simulink model "phm_aug5_powertrain_r2018a"  (R2018a)
settings: Solver=VariableStepAuto  StartTime=0.0  StopTime=750  FixedStep=.01  RelTol=1e-3
InitFcn:
  | addpath fcns;
  | load batteryParams;
  | load motorParams;
  | load ukfBatteryParams;
  | load ukfMotorParams;
undefined symbols (not defined in the file or in its folder): motorParams
libraries: simulink x10
settings Model: Creator=tdarrah  LastModifiedBy=tdarrah
settings SolverCC: ShapePreserveControl=EnableAll  AlgebraicLoopSolver=LineSearch
settings DataIOCC: ReturnWorkspaceOutputs=on
settings SFSimCC: SimUseLocalCustomCode=on
settings RTWCC: RTWUseLocalCustomCode=on

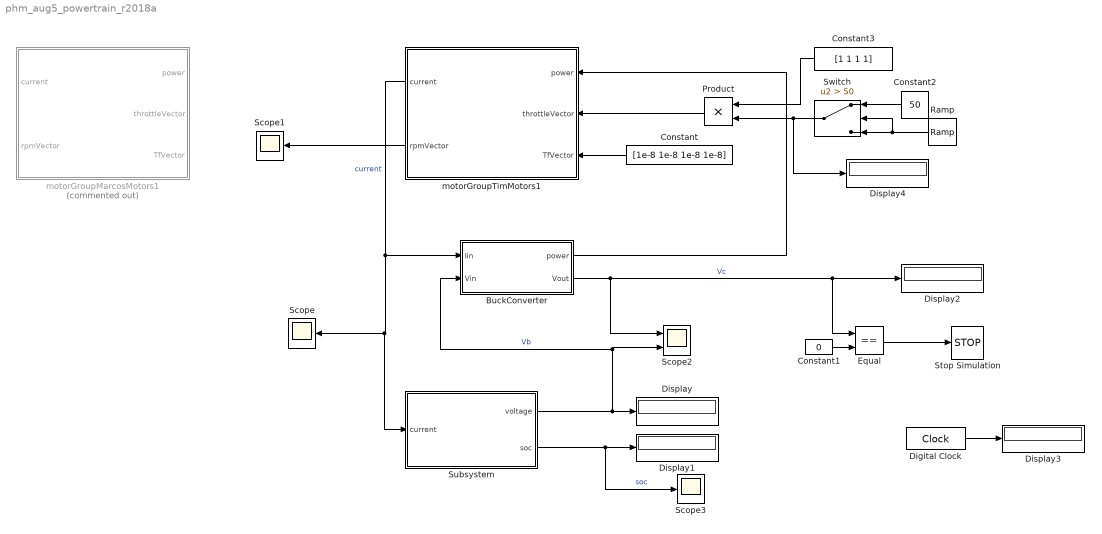
== system phm_aug5_powertrain_r2018a ==
  BuckConverter : Subsystem
  Constant : Constant  Value=[1e-8 1e-8 1e-8 1e-8]
  Constant1 : Constant  Value=0
  Constant2 : Constant  Value=50
  Constant3 : Constant  Value=[1 1 1 1]
  Digital Clock : DigitalClock
      mask Display: disp('Sim Time');
  Display{,1..4} (5 alike) : Display
  Equal : RelationalOperator  Operator===  OutDataTypeStr=boolean  RndMeth=Simplest
  Product : Product
  Ramp : simulink/Sources/Ramp  slope=1  start=0  InitialOutput=0
  Scope : Scope
  Scope1 : Scope
  Scope2 : Scope  NumInputPorts=2
  Scope3 : Scope
  Stop Simulation : Stop
  Subsystem : Subsystem
  Switch : Switch  Criteria=u2 > Threshold  Threshold=50
  motorGroupMarcosMotors1 : Subsystem  Commented=on
  motorGroupTimMotors1 : Subsystem
  wires:
  Subsystem/1(voltage) -> BuckConverter/2(Vin), Scope2/2, Display/1  "Vb"
  Subsystem/2(soc) -> Scope3/1, Display1/1  "soc"
  motorGroupTimMotors1/1(current) -> BuckConverter/1(Iin), Subsystem/1(current), Scope/1  "current"
  BuckConverter/1(power) -> motorGroupTimMotors1/1(power)
  BuckConverter/2(Vout) -> Scope2/1, Equal/1, Display2/1  "Vc"
  Product/1 -> motorGroupTimMotors1/2(throttleVector)
  Constant/1 -> motorGroupTimMotors1/3(TfVector)
  motorGroupTimMotors1/2(rpmVector) -> Scope1/1
  Constant1/1 -> Equal/2
  Equal/1 -> Stop Simulation/1
  Digital Clock/1 -> Display3/1
  Ramp/1 -> Switch/2, Switch/3
  Constant2/1 -> Switch/1
  Constant3/1 -> Product/1
  Switch/1 -> Display4/1, Product/2

== system phm_aug5_powertrain_r2018a/BuckConverter ==
  Iin : Inport
  Vin : Inport  Port=2
  Constant : Constant  Value=0
  Constant2 : Constant  Value=11.4
  If : If  IfExpression=u1 > 10.5
  If Action Subsystem : Subsystem  TreatAsAtomicUnit=on
  If Action Subsystem1 : Subsystem  TreatAsAtomicUnit=on
  Product : Product
  Switch : Switch  Criteria=u2 > Threshold  Threshold=10.5
  power : Outport
  Vout : Outport  Port=2
  wires:
  Product/1 -> power/1
  Iin/1 -> Product/1
  If/1 -> If Action Subsystem/Action
  If/2 -> If Action Subsystem1/Action
  Constant/1 -> If Action Subsystem1/1(In1)
  If Action Subsystem/1(Out1) -> Switch/1
  If Action Subsystem1/1(Out1) -> Switch/3
  Constant2/1 -> If Action Subsystem/1(In1)
  Vin/1 -> Switch/2, If/1
  Switch/1 -> Product/2, Vout/1

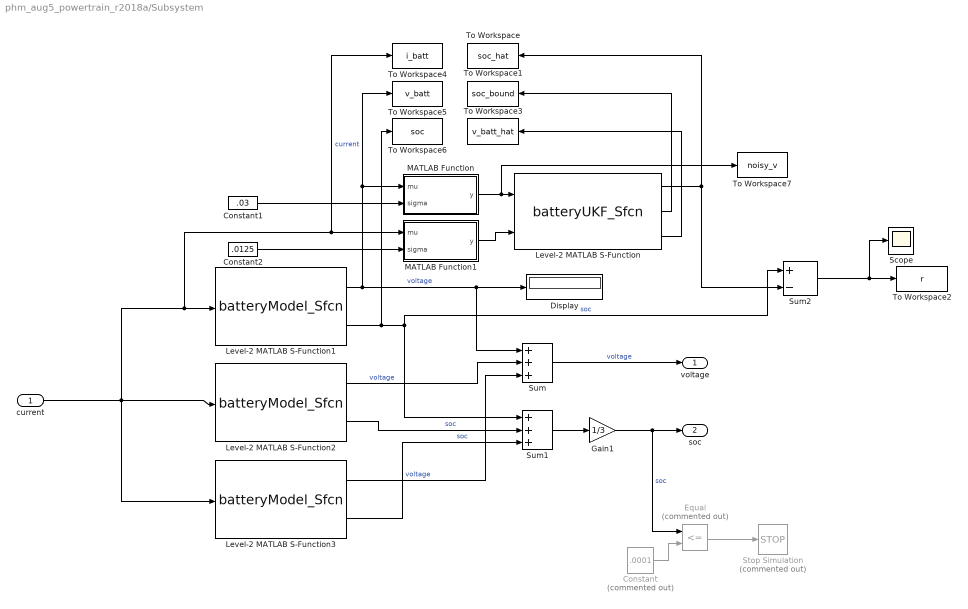
== system phm_aug5_powertrain_r2018a/Subsystem ==
  current : Inport
  Constant : Constant  Commented=on  Value=.0001
  Constant1 : Constant  Value=.03
  Constant2 : Constant  Value=.0125
  Display : Display
  Equal : RelationalOperator  Commented=on  Operator=<=  OutDataTypeStr=boolean  RndMeth=Simplest
  Gain1 : Gain  Gain=1/3
  Level-2 MATLAB S-Function : M-S-Function  FunctionName=batteryUKF_Sfcn  Parameters=batteryParams, batteryParams.dt, ukfBatteryParams
      mask Display:
      | port_label('input', 1, 'voltage');
      | port_label('input', 2, 'current');
      | port_label('output', 1, 'soc_hat');
      | port_label('output', 2, 'soc_bound');
      | port_label('output', 3, 'voltage_hat');
      | 
      | disp("UKF");
  Level-2 MATLAB S-Function1 : M-S-Function  FunctionName=batteryModel_Sfcn  Parameters=batteryParams, batteryParams.dt
      mask Display:
      | port_label('input', 1, 'current');
      | port_label('output', 1, 'voltage');
      | port_label('output', 2, 'soc');
      | 
      | disp("Battery Cell");
  Level-2 MATLAB S-Function2 : M-S-Function  FunctionName=batteryModel_Sfcn  Parameters=batteryParams, batteryParams.dt
      mask Display:
      | port_label('input', 1, 'current');
      | port_label('output', 1, 'voltage');
      | port_label('output', 2, 'soc');
  Level-2 MATLAB S-Function3 : M-S-Function  FunctionName=batteryModel_Sfcn  Parameters=batteryParams, batteryParams.dt
      mask Display:
      | port_label('input', 1, 'current');
      | port_label('output', 1, 'voltage');
      | port_label('output', 2, 'soc');
  MATLAB Function : MATLAB Function  TreatAsAtomicUnit=on
  MATLAB Function1 : MATLAB Function  TreatAsAtomicUnit=on
  Scope : Scope
  Stop Simulation : Stop  Commented=on
  Sum : Sum  Inputs=+++
  Sum1 : Sum  Inputs=+++
  Sum2 : Sum  Inputs=+-
  To Workspace : ToWorkspace  VariableName=soc_hat  SaveFormat=Timeseries  SampleTime=-1
  To Workspace1 : ToWorkspace  VariableName=soc_bound  SaveFormat=Timeseries  SampleTime=-1
  To Workspace2 : ToWorkspace  VariableName=r  SaveFormat=Timeseries  SampleTime=-1
  To Workspace3 : ToWorkspace  VariableName=v_batt_hat  SaveFormat=Timeseries  SampleTime=-1
  To Workspace4 : ToWorkspace  VariableName=i_batt  SaveFormat=Timeseries  SampleTime=-1
  To Workspace5 : ToWorkspace  VariableName=v_batt  SaveFormat=Timeseries  SampleTime=-1
  To Workspace6 : ToWorkspace  VariableName=soc  SaveFormat=Timeseries  SampleTime=-1
  To Workspace7 : ToWorkspace  VariableName=noisy_v  SaveFormat=Timeseries  SampleTime=-1
  voltage : Outport
  soc : Outport  Port=2
  wires:
  Level-2 MATLAB S-Function2/1 -> Sum/2  "voltage"
  Level-2 MATLAB S-Function1/1 -> Display/1, Sum/1, MATLAB Function/1(mu), To Workspace5/1  "voltage"
  Level-2 MATLAB S-Function2/2 -> Sum1/2  "soc"
  Sum1/1 -> Gain1/1
  Gain1/1 -> Equal/1, soc/1  "soc"
  Level-2 MATLAB S-Function1/2 -> To Workspace6/1, Sum2/1, Sum1/1  "soc"
  Level-2 MATLAB S-Function3/2 -> Sum1/3  "soc"
  current/1 -> Level-2 MATLAB S-Function3/1, MATLAB Function1/1(mu), To Workspace4/1, Level-2 MATLAB S-Function1/1, Level-2 MATLAB S-Function2/1  "current"
  Level-2 MATLAB S-Function3/1 -> Sum/3  "voltage"
  Sum/1 -> voltage/1  "voltage"
  Constant/1 -> Equal/2
  Equal/1 -> Stop Simulation/1
  Level-2 MATLAB S-Function/1 -> Sum2/2, To Workspace/1
  Level-2 MATLAB S-Function/2 -> To Workspace1/1
  Sum2/1 -> Scope/1, To Workspace2/1
  Level-2 MATLAB S-Function/3 -> To Workspace3/1
  Constant1/1 -> MATLAB Function/2(sigma)
  MATLAB Function/1(y) -> To Workspace7/1, Level-2 MATLAB S-Function/1
  MATLAB Function1/1(y) -> Level-2 MATLAB S-Function/2
  Constant2/1 -> MATLAB Function1/2(sigma)

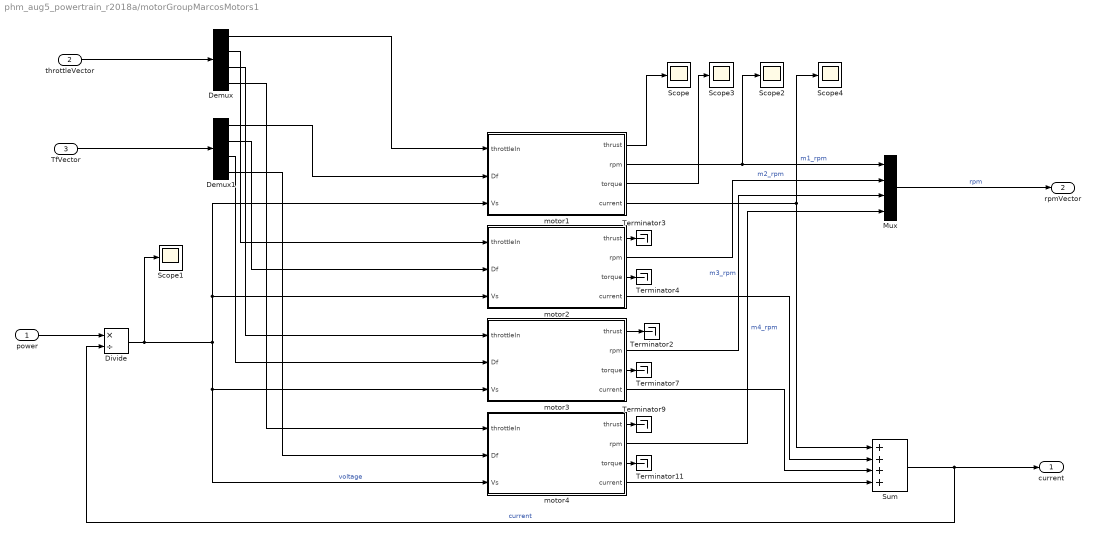
== system phm_aug5_powertrain_r2018a/motorGroupMarcosMotors1 ==
  power : Inport
  throttleVector : Inport  Port=2  PortDimensions=4
  TfVector : Inport  Port=3  PortDimensions=4
  Demux : Demux
  Demux1 : Demux
  Divide : Product  Inputs=*/
  Mux : Mux
  Scope{,1..4} (5 alike) : Scope
  Sum : Sum  Inputs=++++
  Terminator{2..4,7,9,11} (6 alike) : Terminator
  motor1 : Subsystem
  motor2 : Subsystem
  motor3 : Subsystem
  motor4 : Subsystem
  current : Outport
  rpmVector : Outport  Port=2
  wires:
  Demux1/2 -> motor2/2(Df)
  Demux1/4 -> motor4/2(Df)
  Divide/1 -> Scope1/1, motor2/3(Vs), motor1/3(Vs), motor4/3(Vs), motor3/3(Vs)  "voltage"
  Demux1/1 -> motor1/2(Df)
  Sum/1 -> current/1, Divide/2  "current"
  Demux1/3 -> motor3/2(Df)
  motor1/4(current) -> Scope4/1, Sum/1
  power/1 -> Divide/1
  Demux/4 -> motor4/1(throttleIn)
  Demux/3 -> motor3/1(throttleIn)
  Demux/2 -> motor2/1(throttleIn)
  Demux/1 -> motor1/1(throttleIn)
  throttleVector/1 -> Demux/1
  TfVector/1 -> Demux1/1
  motor4/4(current) -> Sum/4
  motor3/4(current) -> Sum/3
  motor2/4(current) -> Sum/2
  motor4/2(rpm) -> Mux/4  "m4_rpm"
  motor3/2(rpm) -> Mux/3  "m3_rpm"
  motor2/2(rpm) -> Mux/2  "m2_rpm"
  motor1/2(rpm) -> Scope2/1, Mux/1  "m1_rpm"
  Mux/1 -> rpmVector/1  "rpm"
  motor1/1(thrust) -> Scope/1
  motor4/3(torque) -> Terminator11/1
  motor1/3(torque) -> Scope3/1
  motor2/3(torque) -> Terminator4/1
  motor3/3(torque) -> Terminator7/1
  motor4/1(thrust) -> Terminator9/1
  motor3/1(thrust) -> Terminator2/1
  motor2/1(thrust) -> Terminator3/1

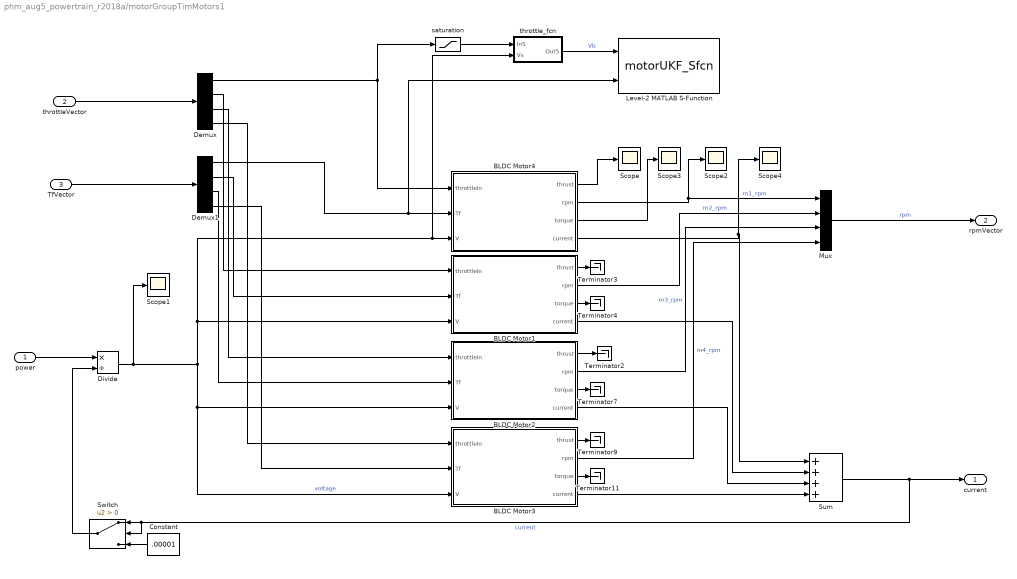
== system phm_aug5_powertrain_r2018a/motorGroupTimMotors1 ==
  power : Inport
  throttleVector : Inport  Port=2  PortDimensions=4
  TfVector : Inport  Port=3  PortDimensions=4
  BLDC Motor1 : Subsystem
  BLDC Motor2 : Subsystem
  BLDC Motor3 : Subsystem
  BLDC Motor4 : Subsystem
  Constant : Constant  Value=.00001
  Demux : Demux
  Demux1 : Demux
  Divide : Product  Inputs=*/
  Level-2 MATLAB S-Function : M-S-Function  FunctionName=motorUKF_Sfcn  Parameters=motorParams, ukfMotorParams
      mask Display:
      | port_label('input', 1, 'voltage');
      | port_label('input', 2, 'friction');
      | port_label('output', 1, 'rpm');
      | port_label('output', 2, 'current');
      | port_label('output', 3, 'torque');
      | port_label('output', 4, 'bounds');
      | disp("Motor UKF");
  Mux : Mux
  Scope{,1..4} (5 alike) : Scope
  Sum : Sum  Inputs=++++
  Switch : Switch  Criteria=u2 > Threshold
  Terminator{2..4,7,9,11} (6 alike) : Terminator
  saturation : Saturate  UpperLimit=100  LowerLimit=0
  throttle_fcn : Subsystem
  current : Outport
  rpmVector : Outport  Port=2
  wires:
  Demux1/2 -> BLDC Motor1/2(Tf)
  Demux1/4 -> BLDC Motor3/2(Tf)
  Divide/1 -> Scope1/1, BLDC Motor1/3(V), throttle_fcn/2(Vs), BLDC Motor4/3(V), BLDC Motor3/3(V), BLDC Motor2/3(V)  "voltage"
  Demux1/1 -> Level-2 MATLAB S-Function/2, BLDC Motor4/2(Tf)
  Sum/1 -> Switch/2, Switch/1, current/1  "current"
  Demux1/3 -> BLDC Motor2/2(Tf)
  BLDC Motor4/4(current) -> Scope4/1, Sum/1
  power/1 -> Divide/1
  Demux/4 -> BLDC Motor3/1(throttleIn)
  Demux/3 -> BLDC Motor2/1(throttleIn)
  Demux/2 -> BLDC Motor1/1(throttleIn)
  Demux/1 -> saturation/1, BLDC Motor4/1(throttleIn)
  throttleVector/1 -> Demux/1
  TfVector/1 -> Demux1/1
  BLDC Motor3/4(current) -> Sum/4
  BLDC Motor2/4(current) -> Sum/3
  BLDC Motor1/4(current) -> Sum/2
  BLDC Motor3/2(rpm) -> Mux/4  "m4_rpm"
  BLDC Motor2/2(rpm) -> Mux/3  "m3_rpm"
  BLDC Motor1/2(rpm) -> Mux/2  "m2_rpm"
  BLDC Motor4/2(rpm) -> Scope2/1, Mux/1  "m1_rpm"
  Mux/1 -> rpmVector/1  "rpm"
  BLDC Motor4/1(thrust) -> Scope/1
  BLDC Motor3/3(torque) -> Terminator11/1
  BLDC Motor4/3(torque) -> Scope3/1
  BLDC Motor1/3(torque) -> Terminator4/1
  BLDC Motor2/3(torque) -> Terminator7/1
  BLDC Motor3/1(thrust) -> Terminator9/1
  BLDC Motor2/1(thrust) -> Terminator2/1
  BLDC Motor1/1(thrust) -> Terminator3/1
  Switch/1 -> Divide/2
  Constant/1 -> Switch/3
  throttle_fcn/1(Out5) -> Level-2 MATLAB S-Function/1  "Vb"
  saturation/1 -> throttle_fcn/1(In5)

== system phm_aug5_powertrain_r2018a/BuckConverter/If Action Subsystem ==
  In1 : Inport
  Action Port : ActionPort
  Out1 : Outport
  wires:
  In1/1 -> Out1/1

== system phm_aug5_powertrain_r2018a/BuckConverter/If Action Subsystem1 ==
  In1 : Inport
  Action Port : ActionPort
  Out1 : Outport
  wires:
  In1/1 -> Out1/1

== system phm_aug5_powertrain_r2018a/motorGroupMarcosMotors1/motor1 ==
  note: Throttle cutoff can simulate the fact that the motor doesn't
      | spin until a minimum throttle point is reached. This introduces
      | a jump discontinuity in low throttle performance.
  note: These saturations model a SIGNAL LIMITATION.
      | Other intentional control saturations might be introduced in the
      | control loop to achieve better stability and consistency.
  throttleIn : Inport
  Df : Inport  Port=2
  Vs : Inport  Port=3
  Scope : Scope
  Signal_Saturation_4 : Saturate  UpperLimit=100  LowerLimit=0
  Throttle To RPM Gain and Cutoff_8 : Subsystem
  motorRotor4 : Subsystem
  thrust : Outport
  rpm : Outport  Port=2
  torque : Outport  Port=3
  current : Outport  Port=4
  wires:
  Throttle To RPM Gain and Cutoff_8/1(Out5) -> motorRotor4/1(V), Scope/1
  motorRotor4/4(current) -> current/1
  motorRotor4/2(rpm) -> rpm/1
  throttleIn/1 -> Signal_Saturation_4/1
  motorRotor4/3(torque) -> torque/1
  motorRotor4/1(thrust) -> thrust/1
  Signal_Saturation_4/1 -> Throttle To RPM Gain and Cutoff_8/1(In5)
  Df/1 -> motorRotor4/2(Df)
  Vs/1 -> Throttle To RPM Gain and Cutoff_8/2(Vs)

== system phm_aug5_powertrain_r2018a/motorGroupMarcosMotors1/motor2 ==
  note: Throttle cutoff can simulate the fact that the motor doesn't
      | spin until a minimum throttle point is reached. This introduces
      | a jump discontinuity in low throttle performance.
  note: These saturations model a SIGNAL LIMITATION.
      | Other intentional control saturations might be introduced in the
      | control loop to achieve better stability and consistency.
  throttleIn : Inport
  Df : Inport  Port=2
  Vs : Inport  Port=3
  Scope : Scope
  Signal_Saturation_4 : Saturate  UpperLimit=100  LowerLimit=0
  Throttle To RPM Gain and Cutoff_8 : Subsystem
  motorRotor4 : Subsystem
  thrust : Outport
  rpm : Outport  Port=2
  torque : Outport  Port=3
  current : Outport  Port=4
  wires:
  Throttle To RPM Gain and Cutoff_8/1(Out5) -> motorRotor4/1(V), Scope/1
  motorRotor4/4(current) -> current/1
  motorRotor4/2(rpm) -> rpm/1
  throttleIn/1 -> Signal_Saturation_4/1
  motorRotor4/3(torque) -> torque/1
  motorRotor4/1(thrust) -> thrust/1
  Signal_Saturation_4/1 -> Throttle To RPM Gain and Cutoff_8/1(In5)
  Df/1 -> motorRotor4/2(Df)
  Vs/1 -> Throttle To RPM Gain and Cutoff_8/2(Vs)

== system phm_aug5_powertrain_r2018a/motorGroupMarcosMotors1/motor3 ==
  note: Throttle cutoff can simulate the fact that the motor doesn't
      | spin until a minimum throttle point is reached. This introduces
      | a jump discontinuity in low throttle performance.
  note: These saturations model a SIGNAL LIMITATION.
      | Other intentional control saturations might be introduced in the
      | control loop to achieve better stability and consistency.
  throttleIn : Inport
  Df : Inport  Port=2
  Vs : Inport  Port=3
  Scope : Scope
  Signal_Saturation_4 : Saturate  UpperLimit=100  LowerLimit=0
  Throttle To RPM Gain and Cutoff_8 : Subsystem
  motorRotor4 : Subsystem
  thrust : Outport
  rpm : Outport  Port=2
  torque : Outport  Port=3
  current : Outport  Port=4
  wires:
  Throttle To RPM Gain and Cutoff_8/1(Out5) -> motorRotor4/1(V), Scope/1
  motorRotor4/4(current) -> current/1
  motorRotor4/2(rpm) -> rpm/1
  throttleIn/1 -> Signal_Saturation_4/1
  motorRotor4/3(torque) -> torque/1
  motorRotor4/1(thrust) -> thrust/1
  Signal_Saturation_4/1 -> Throttle To RPM Gain and Cutoff_8/1(In5)
  Df/1 -> motorRotor4/2(Df)
  Vs/1 -> Throttle To RPM Gain and Cutoff_8/2(Vs)

== system phm_aug5_powertrain_r2018a/motorGroupMarcosMotors1/motor4 ==
  note: Throttle cutoff can simulate the fact that the motor doesn't
      | spin until a minimum throttle point is reached. This introduces
      | a jump discontinuity in low throttle performance.
  note: These saturations model a SIGNAL LIMITATION.
      | Other intentional control saturations might be introduced in the
      | control loop to achieve better stability and consistency.
  throttleIn : Inport
  Df : Inport  Port=2
  Vs : Inport  Port=3
  Scope : Scope
  Signal_Saturation_4 : Saturate  UpperLimit=100  LowerLimit=0
  Throttle To RPM Gain and Cutoff_8 : Subsystem
  motorRotor4 : Subsystem
  thrust : Outport
  rpm : Outport  Port=2
  torque : Outport  Port=3
  current : Outport  Port=4
  wires:
  Throttle To RPM Gain and Cutoff_8/1(Out5) -> motorRotor4/1(V), Scope/1
  motorRotor4/4(current) -> current/1
  motorRotor4/2(rpm) -> rpm/1
  throttleIn/1 -> Signal_Saturation_4/1
  motorRotor4/3(torque) -> torque/1
  motorRotor4/1(thrust) -> thrust/1
  Signal_Saturation_4/1 -> Throttle To RPM Gain and Cutoff_8/1(In5)
  Df/1 -> motorRotor4/2(Df)
  Vs/1 -> Throttle To RPM Gain and Cutoff_8/2(Vs)

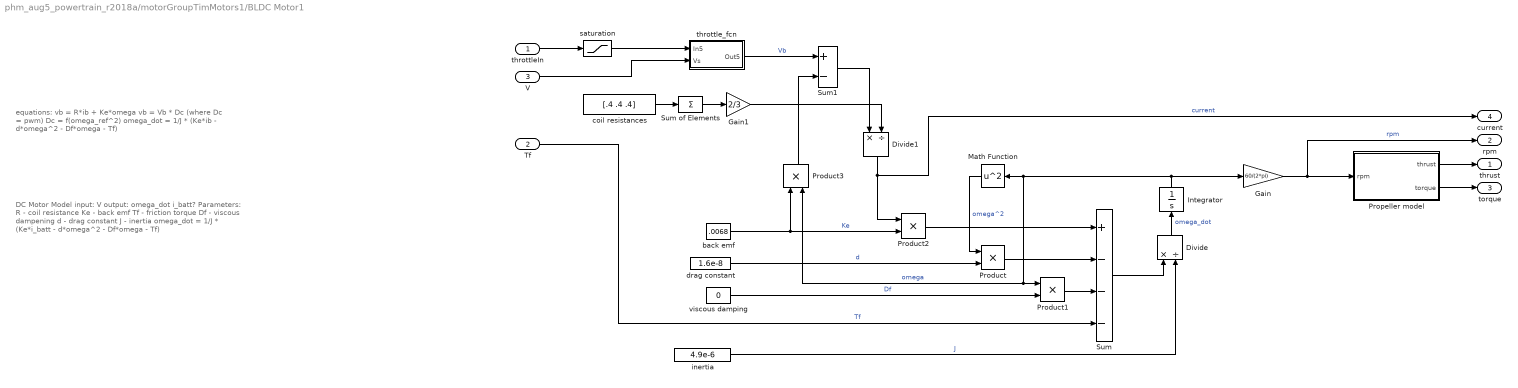
== system phm_aug5_powertrain_r2018a/motorGroupTimMotors1/BLDC Motor1 ==
  note: DC Motor Model
      |
      | input:
      | V
      |
      | output:
      | omega_dot
      | i_batt?
      |
      |
      | Parameters:
      | R   - coil resistance
      | Ke - back emf
      | Tf  - friction torque
      | Df  - viscous dampening
      | d   - drag constant
      | J   - inertia
      |
      | omega_dot = 1/J * (Ke*i_batt - d*omega^2 - Df*omega - Tf)
  note: equations:
      |
      | vb = R*ib + Ke*omega
      | vb = Vb * Dc  (where Dc = pwm)
      | Dc = f(omega_ref^2)
      |
      | omega_dot = 1/J * (Ke*ib - d*omega^2 - Df*omega - Tf)
  throttleIn : Inport
  Tf : Inport  Port=2
  V : Inport  Port=3
  Divide : Product  Inputs=*/
  Divide1 : Product  Inputs=*/
  Gain : Gain  Gain=60/(2*pi)
  Gain1 : Gain  Gain=2/3
  Integrator : Integrator
  Math Function : Math  Operator=square  SaturateOnIntegerOverflow=on
  Product{,1..3} (4 alike) : Product
  "Propeller model " : MATLAB Function  TreatAsAtomicUnit=on
  Sum : Sum  Inputs=+---
  Sum of Elements : Sum  Inputs=+
  Sum1 : Sum  Inputs=+-
  back emf : Constant  Value=.0068
  coil resistances : Constant  Value=[.4 .4 .4]
  drag constant : Constant  Value=1.6e-8
  inertia : Constant  Value=4.9e-6
  saturation : Saturate  UpperLimit=100  LowerLimit=0
  throttle_fcn : Subsystem
  viscous damping : Constant  Value=0
  thrust : Outport
  rpm : Outport  Port=2
  torque : Outport  Port=3
  current : Outport  Port=4
  wires:
  Divide/1 -> Integrator/1  "omega_dot"
  Integrator/1 -> Gain/1, Math Function/1, Product1/1, Product3/2  "omega"
  Gain/1 -> "Propeller model "/1(rpm), rpm/1  "rpm"
  inertia/1 -> Divide/2  "J"
  drag constant/1 -> Product/2  "d"
  Math Function/1 -> Product/1  "omega^2"
  viscous damping/1 -> Product1/2  "Df"
  Tf/1 -> Sum/4  "Tf"
  back emf/1 -> Product3/1, Product2/2  "Ke"
  Product2/1 -> Sum/1
  Divide1/1 -> current/1, Product2/1  "current"
  V/1 -> throttle_fcn/2(Vs)
  Product3/1 -> Sum1/2
  Sum1/1 -> Divide1/1
  Gain1/1 -> Divide1/2
  "Propeller model "/1(thrust) -> thrust/1
  "Propeller model "/2(torque) -> torque/1
  Product1/1 -> Sum/3
  Product/1 -> Sum/2
  Sum/1 -> Divide/1
  coil resistances/1 -> Sum of Elements/1
  Sum of Elements/1 -> Gain1/1
  throttleIn/1 -> saturation/1
  throttle_fcn/1(Out5) -> Sum1/1  "Vb"
  saturation/1 -> throttle_fcn/1(In5)

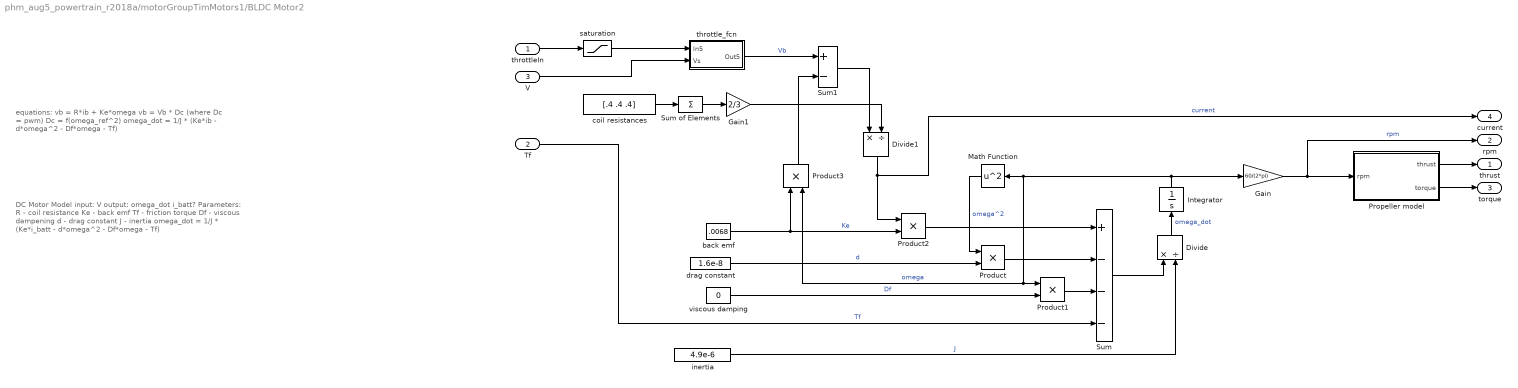
== system phm_aug5_powertrain_r2018a/motorGroupTimMotors1/BLDC Motor2 ==
  note: DC Motor Model
      |
      | input:
      | V
      |
      | output:
      | omega_dot
      | i_batt?
      |
      |
      | Parameters:
      | R   - coil resistance
      | Ke - back emf
      | Tf  - friction torque
      | Df  - viscous dampening
      | d   - drag constant
      | J   - inertia
      |
      | omega_dot = 1/J * (Ke*i_batt - d*omega^2 - Df*omega - Tf)
  note: equations:
      |
      | vb = R*ib + Ke*omega
      | vb = Vb * Dc  (where Dc = pwm)
      | Dc = f(omega_ref^2)
      |
      | omega_dot = 1/J * (Ke*ib - d*omega^2 - Df*omega - Tf)
  throttleIn : Inport
  Tf : Inport  Port=2
  V : Inport  Port=3
  Divide : Product  Inputs=*/
  Divide1 : Product  Inputs=*/
  Gain : Gain  Gain=60/(2*pi)
  Gain1 : Gain  Gain=2/3
  Integrator : Integrator
  Math Function : Math  Operator=square  SaturateOnIntegerOverflow=on
  Product{,1..3} (4 alike) : Product
  "Propeller model " : MATLAB Function  TreatAsAtomicUnit=on
  Sum : Sum  Inputs=+---
  Sum of Elements : Sum  Inputs=+
  Sum1 : Sum  Inputs=+-
  back emf : Constant  Value=.0068
  coil resistances : Constant  Value=[.4 .4 .4]
  drag constant : Constant  Value=1.6e-8
  inertia : Constant  Value=4.9e-6
  saturation : Saturate  UpperLimit=100  LowerLimit=0
  throttle_fcn : Subsystem
  viscous damping : Constant  Value=0
  thrust : Outport
  rpm : Outport  Port=2
  torque : Outport  Port=3
  current : Outport  Port=4
  wires:
  Divide/1 -> Integrator/1  "omega_dot"
  Integrator/1 -> Gain/1, Math Function/1, Product1/1, Product3/2  "omega"
  Gain/1 -> "Propeller model "/1(rpm), rpm/1  "rpm"
  inertia/1 -> Divide/2  "J"
  drag constant/1 -> Product/2  "d"
  Math Function/1 -> Product/1  "omega^2"
  viscous damping/1 -> Product1/2  "Df"
  Tf/1 -> Sum/4  "Tf"
  back emf/1 -> Product3/1, Product2/2  "Ke"
  Product2/1 -> Sum/1
  Divide1/1 -> current/1, Product2/1  "current"
  V/1 -> throttle_fcn/2(Vs)
  Product3/1 -> Sum1/2
  Sum1/1 -> Divide1/1
  Gain1/1 -> Divide1/2
  "Propeller model "/1(thrust) -> thrust/1
  "Propeller model "/2(torque) -> torque/1
  Product1/1 -> Sum/3
  Product/1 -> Sum/2
  Sum/1 -> Divide/1
  coil resistances/1 -> Sum of Elements/1
  Sum of Elements/1 -> Gain1/1
  throttleIn/1 -> saturation/1
  throttle_fcn/1(Out5) -> Sum1/1  "Vb"
  saturation/1 -> throttle_fcn/1(In5)

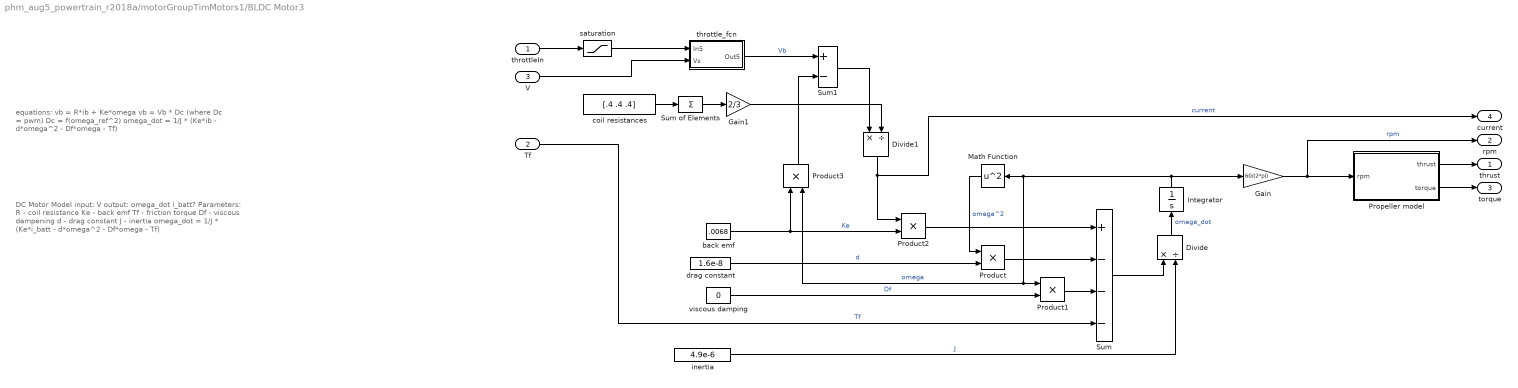
== system phm_aug5_powertrain_r2018a/motorGroupTimMotors1/BLDC Motor3 ==
  note: DC Motor Model
      |
      | input:
      | V
      |
      | output:
      | omega_dot
      | i_batt?
      |
      |
      | Parameters:
      | R   - coil resistance
      | Ke - back emf
      | Tf  - friction torque
      | Df  - viscous dampening
      | d   - drag constant
      | J   - inertia
      |
      | omega_dot = 1/J * (Ke*i_batt - d*omega^2 - Df*omega - Tf)
  note: equations:
      |
      | vb = R*ib + Ke*omega
      | vb = Vb * Dc  (where Dc = pwm)
      | Dc = f(omega_ref^2)
      |
      | omega_dot = 1/J * (Ke*ib - d*omega^2 - Df*omega - Tf)
  throttleIn : Inport
  Tf : Inport  Port=2
  V : Inport  Port=3
  Divide : Product  Inputs=*/
  Divide1 : Product  Inputs=*/
  Gain : Gain  Gain=60/(2*pi)
  Gain1 : Gain  Gain=2/3
  Integrator : Integrator
  Math Function : Math  Operator=square  SaturateOnIntegerOverflow=on
  Product{,1..3} (4 alike) : Product
  "Propeller model " : MATLAB Function  TreatAsAtomicUnit=on
  Sum : Sum  Inputs=+---
  Sum of Elements : Sum  Inputs=+
  Sum1 : Sum  Inputs=+-
  back emf : Constant  Value=.0068
  coil resistances : Constant  Value=[.4 .4 .4]
  drag constant : Constant  Value=1.6e-8
  inertia : Constant  Value=4.9e-6
  saturation : Saturate  UpperLimit=100  LowerLimit=0
  throttle_fcn : Subsystem
  viscous damping : Constant  Value=0
  thrust : Outport
  rpm : Outport  Port=2
  torque : Outport  Port=3
  current : Outport  Port=4
  wires:
  Divide/1 -> Integrator/1  "omega_dot"
  Integrator/1 -> Gain/1, Math Function/1, Product1/1, Product3/2  "omega"
  Gain/1 -> "Propeller model "/1(rpm), rpm/1  "rpm"
  inertia/1 -> Divide/2  "J"
  drag constant/1 -> Product/2  "d"
  Math Function/1 -> Product/1  "omega^2"
  viscous damping/1 -> Product1/2  "Df"
  Tf/1 -> Sum/4  "Tf"
  back emf/1 -> Product3/1, Product2/2  "Ke"
  Product2/1 -> Sum/1
  Divide1/1 -> current/1, Product2/1  "current"
  V/1 -> throttle_fcn/2(Vs)
  Product3/1 -> Sum1/2
  Sum1/1 -> Divide1/1
  Gain1/1 -> Divide1/2
  "Propeller model "/1(thrust) -> thrust/1
  "Propeller model "/2(torque) -> torque/1
  Product1/1 -> Sum/3
  Product/1 -> Sum/2
  Sum/1 -> Divide/1
  coil resistances/1 -> Sum of Elements/1
  Sum of Elements/1 -> Gain1/1
  throttleIn/1 -> saturation/1
  throttle_fcn/1(Out5) -> Sum1/1  "Vb"
  saturation/1 -> throttle_fcn/1(In5)

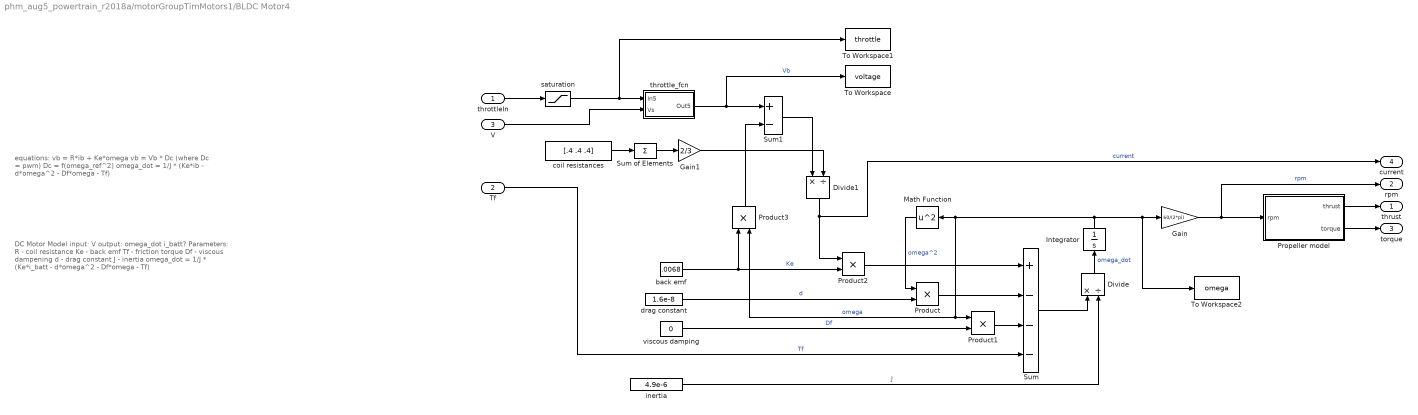
== system phm_aug5_powertrain_r2018a/motorGroupTimMotors1/BLDC Motor4 ==
  note: DC Motor Model
      |
      | input:
      | V
      |
      | output:
      | omega_dot
      | i_batt?
      |
      |
      | Parameters:
      | R   - coil resistance
      | Ke - back emf
      | Tf  - friction torque
      | Df  - viscous dampening
      | d   - drag constant
      | J   - inertia
      |
      | omega_dot = 1/J * (Ke*i_batt - d*omega^2 - Df*omega - Tf)
  note: equations:
      |
      | vb = R*ib + Ke*omega
      | vb = Vb * Dc  (where Dc = pwm)
      | Dc = f(omega_ref^2)
      |
      | omega_dot = 1/J * (Ke*ib - d*omega^2 - Df*omega - Tf)
  throttleIn : Inport
  Tf : Inport  Port=2
  V : Inport  Port=3
  Divide : Product  Inputs=*/
  Divide1 : Product  Inputs=*/
  Gain : Gain  Gain=60/(2*pi)
  Gain1 : Gain  Gain=2/3
  Integrator : Integrator
  Math Function : Math  Operator=square  SaturateOnIntegerOverflow=on
  Product{,1..3} (4 alike) : Product
  "Propeller model " : MATLAB Function  TreatAsAtomicUnit=on
  Sum : Sum  Inputs=+---
  Sum of Elements : Sum  Inputs=+
  Sum1 : Sum  Inputs=+-
  To Workspace : ToWorkspace  VariableName=voltage  SaveFormat=Timeseries  SampleTime=-1
  To Workspace1 : ToWorkspace  VariableName=throttle  SaveFormat=Timeseries  SampleTime=-1
  To Workspace2 : ToWorkspace  VariableName=omega  SaveFormat=Timeseries  SampleTime=-1
  back emf : Constant  Value=.0068
  coil resistances : Constant  Value=[.4 .4 .4]
  drag constant : Constant  Value=1.6e-8
  inertia : Constant  Value=4.9e-6
  saturation : Saturate  UpperLimit=100  LowerLimit=0
  throttle_fcn : Subsystem
  viscous damping : Constant  Value=0
  thrust : Outport
  rpm : Outport  Port=2
  torque : Outport  Port=3
  current : Outport  Port=4
  wires:
  Divide/1 -> Integrator/1  "omega_dot"
  Integrator/1 -> To Workspace2/1, Gain/1, Math Function/1, Product1/1, Product3/2  "omega"
  Gain/1 -> "Propeller model "/1(rpm), rpm/1  "rpm"
  inertia/1 -> Divide/2  "J"
  drag constant/1 -> Product/2  "d"
  Math Function/1 -> Product/1  "omega^2"
  viscous damping/1 -> Product1/2  "Df"
  Tf/1 -> Sum/4  "Tf"
  back emf/1 -> Product3/1, Product2/2  "Ke"
  Product2/1 -> Sum/1
  Divide1/1 -> current/1, Product2/1  "current"
  V/1 -> throttle_fcn/2(Vs)
  Product3/1 -> Sum1/2
  Sum1/1 -> Divide1/1
  Gain1/1 -> Divide1/2
  "Propeller model "/1(thrust) -> thrust/1
  "Propeller model "/2(torque) -> torque/1
  Product1/1 -> Sum/3
  Product/1 -> Sum/2
  Sum/1 -> Divide/1
  coil resistances/1 -> Sum of Elements/1
  Sum of Elements/1 -> Gain1/1
  throttleIn/1 -> saturation/1
  throttle_fcn/1(Out5) -> To Workspace/1, Sum1/1  "Vb"
  saturation/1 -> To Workspace1/1, throttle_fcn/1(In5)

== system phm_aug5_powertrain_r2018a/motorGroupTimMotors1/throttle_fcn ==
  note: Output equals linearly scaled RPM
      | for given throttle input if throttle input >=Throttle Cuttoff (minThr)
      | else output is zero.
  In5 : Inport
  Vs : Inport  Port=2
  Gain : Gain  Gain=.01
  Minimum Throttle Cutoff : simulink/Logic and Bit Operations/Compare To Constant  relop=>=  const=5  OutDataTypeStr=uint8
  Product : Product
  Product2 : Product
  Out5 : Outport
  wires:
  Minimum Throttle Cutoff/1 -> Product/2
  Product/1 -> Out5/1
  In5/1 -> Gain/1, Minimum Throttle Cutoff/1
  Gain/1 -> Product2/2
  Product2/1 -> Product/1
  Vs/1 -> Product2/1

== system phm_aug5_powertrain_r2018a/motorGroupMarcosMotors1/motor1/Throttle To RPM Gain and Cutoff_8 ==
  note: Output equals linearly scaled RPM
      | for given throttle input if throttle input >=Throttle Cuttoff (minThr)
      | else output is zero.
  In5 : Inport
  Vs : Inport  Port=2
  Gain : Gain  Gain=.01
  Minimum Throttle Cutoff : simulink/Logic and Bit Operations/Compare To Constant  relop=>=  const=5  OutDataTypeStr=uint8
  Product : Product
  Product2 : Product
  Out5 : Outport
  wires:
  Minimum Throttle Cutoff/1 -> Product/2
  Product/1 -> Out5/1
  In5/1 -> Gain/1, Minimum Throttle Cutoff/1
  Gain/1 -> Product2/2
  Product2/1 -> Product/1
  Vs/1 -> Product2/1

== system phm_aug5_powertrain_r2018a/motorGroupMarcosMotors1/motor1/motorRotor4 ==
  V : Inport
  Df : Inport  Port=2
  Electrical part : Subsystem
  Mechanical part : Subsystem
  thrust : Outport
  rpm : Outport  Port=2
  torque : Outport  Port=3
  current : Outport  Port=4
  wires:
  V/1 -> Electrical part/1(Vin)
  Mechanical part/2(Thrust) -> thrust/1
  Electrical part/1(Electrical Torque) -> Mechanical part/2(Electrical Torque)
  Mechanical part/4(Torque) -> torque/1
  Mechanical part/1(w angular speed) -> Electrical part/2(w angular speed)
  Df/1 -> Mechanical part/1(dynamicFriction)
  Electrical part/2(current) -> current/1
  Mechanical part/3(rpm) -> rpm/1

== system phm_aug5_powertrain_r2018a/motorGroupMarcosMotors1/motor2/Throttle To RPM Gain and Cutoff_8 ==
  note: Output equals linearly scaled RPM
      | for given throttle input if throttle input >=Throttle Cuttoff (minThr)
      | else output is zero.
  In5 : Inport
  Vs : Inport  Port=2
  Gain : Gain  Gain=.01
  Minimum Throttle Cutoff : simulink/Logic and Bit Operations/Compare To Constant  relop=>=  const=5  OutDataTypeStr=uint8
  Product : Product
  Product2 : Product
  Out5 : Outport
  wires:
  Minimum Throttle Cutoff/1 -> Product/2
  Product/1 -> Out5/1
  In5/1 -> Gain/1, Minimum Throttle Cutoff/1
  Gain/1 -> Product2/2
  Product2/1 -> Product/1
  Vs/1 -> Product2/1

== system phm_aug5_powertrain_r2018a/motorGroupMarcosMotors1/motor2/motorRotor4 ==
  V : Inport
  Df : Inport  Port=2
  Electrical part : Subsystem
  Mechanical part : Subsystem
  thrust : Outport
  rpm : Outport  Port=2
  torque : Outport  Port=3
  current : Outport  Port=4
  wires:
  V/1 -> Electrical part/1(Vin)
  Mechanical part/2(Thrust) -> thrust/1
  Electrical part/1(Electrical Torque) -> Mechanical part/2(Electrical Torque)
  Mechanical part/4(Torque) -> torque/1
  Mechanical part/1(w angular speed) -> Electrical part/2(w angular speed)
  Df/1 -> Mechanical part/1(dynamicFriction)
  Electrical part/2(current) -> current/1
  Mechanical part/3(rpm) -> rpm/1

== system phm_aug5_powertrain_r2018a/motorGroupMarcosMotors1/motor3/Throttle To RPM Gain and Cutoff_8 ==
  note: Output equals linearly scaled RPM
      | for given throttle input if throttle input >=Throttle Cuttoff (minThr)
      | else output is zero.
  In5 : Inport
  Vs : Inport  Port=2
  Gain : Gain  Gain=.01
  Minimum Throttle Cutoff : simulink/Logic and Bit Operations/Compare To Constant  relop=>=  const=5  OutDataTypeStr=uint8
  Product : Product
  Product2 : Product
  Out5 : Outport
  wires:
  Minimum Throttle Cutoff/1 -> Product/2
  Product/1 -> Out5/1
  In5/1 -> Gain/1, Minimum Throttle Cutoff/1
  Gain/1 -> Product2/2
  Product2/1 -> Product/1
  Vs/1 -> Product2/1

== system phm_aug5_powertrain_r2018a/motorGroupMarcosMotors1/motor3/motorRotor4 ==
  V : Inport
  Df : Inport  Port=2
  Electrical part : Subsystem
  Mechanical part : Subsystem
  thrust : Outport
  rpm : Outport  Port=2
  torque : Outport  Port=3
  current : Outport  Port=4
  wires:
  V/1 -> Electrical part/1(Vin)
  Mechanical part/2(Thrust) -> thrust/1
  Electrical part/1(Electrical Torque) -> Mechanical part/2(Electrical Torque)
  Mechanical part/4(Torque) -> torque/1
  Mechanical part/1(w angular speed) -> Electrical part/2(w angular speed)
  Df/1 -> Mechanical part/1(dynamicFriction)
  Electrical part/2(current) -> current/1
  Mechanical part/3(rpm) -> rpm/1

== system phm_aug5_powertrain_r2018a/motorGroupMarcosMotors1/motor4/Throttle To RPM Gain and Cutoff_8 ==
  note: Output equals linearly scaled RPM
      | for given throttle input if throttle input >=Throttle Cuttoff (minThr)
      | else output is zero.
  In5 : Inport
  Vs : Inport  Port=2
  Gain : Gain  Gain=.01
  Minimum Throttle Cutoff : simulink/Logic and Bit Operations/Compare To Constant  relop=>=  const=5  OutDataTypeStr=uint8
  Product : Product
  Product2 : Product
  Out5 : Outport
  wires:
  Minimum Throttle Cutoff/1 -> Product/2
  Product/1 -> Out5/1
  In5/1 -> Gain/1, Minimum Throttle Cutoff/1
  Gain/1 -> Product2/2
  Product2/1 -> Product/1
  Vs/1 -> Product2/1

== system phm_aug5_powertrain_r2018a/motorGroupMarcosMotors1/motor4/motorRotor4 ==
  V : Inport
  Df : Inport  Port=2
  Electrical part : Subsystem
  Mechanical part : Subsystem
  thrust : Outport
  rpm : Outport  Port=2
  torque : Outport  Port=3
  current : Outport  Port=4
  wires:
  V/1 -> Electrical part/1(Vin)
  Mechanical part/2(Thrust) -> thrust/1
  Electrical part/1(Electrical Torque) -> Mechanical part/2(Electrical Torque)
  Mechanical part/4(Torque) -> torque/1
  Mechanical part/1(w angular speed) -> Electrical part/2(w angular speed)
  Df/1 -> Mechanical part/1(dynamicFriction)
  Electrical part/2(current) -> current/1
  Mechanical part/3(rpm) -> rpm/1

== system phm_aug5_powertrain_r2018a/motorGroupTimMotors1/BLDC Motor1/throttle_fcn ==
  note: Output equals linearly scaled RPM
      | for given throttle input if throttle input >=Throttle Cuttoff (minThr)
      | else output is zero.
  In5 : Inport
  Vs : Inport  Port=2
  Gain : Gain  Gain=.01
  Minimum Throttle Cutoff : simulink/Logic and Bit Operations/Compare To Constant  relop=>=  const=5  OutDataTypeStr=uint8
  Product : Product
  Product2 : Product  OutDataTypeStr=double
  Out5 : Outport
  wires:
  Minimum Throttle Cutoff/1 -> Product/2
  Product/1 -> Out5/1
  In5/1 -> Gain/1, Minimum Throttle Cutoff/1
  Gain/1 -> Product2/2
  Product2/1 -> Product/1
  Vs/1 -> Product2/1

== system phm_aug5_powertrain_r2018a/motorGroupTimMotors1/BLDC Motor2/throttle_fcn ==
  note: Output equals linearly scaled RPM
      | for given throttle input if throttle input >=Throttle Cuttoff (minThr)
      | else output is zero.
  In5 : Inport
  Vs : Inport  Port=2
  Gain : Gain  Gain=.01
  Minimum Throttle Cutoff : simulink/Logic and Bit Operations/Compare To Constant  relop=>=  const=5  OutDataTypeStr=uint8
  Product : Product
  Product2 : Product  OutDataTypeStr=double
  Out5 : Outport
  wires:
  Minimum Throttle Cutoff/1 -> Product/2
  Product/1 -> Out5/1
  In5/1 -> Gain/1, Minimum Throttle Cutoff/1
  Gain/1 -> Product2/2
  Product2/1 -> Product/1
  Vs/1 -> Product2/1

== system phm_aug5_powertrain_r2018a/motorGroupTimMotors1/BLDC Motor3/throttle_fcn ==
  note: Output equals linearly scaled RPM
      | for given throttle input if throttle input >=Throttle Cuttoff (minThr)
      | else output is zero.
  In5 : Inport
  Vs : Inport  Port=2
  Gain : Gain  Gain=.01
  Minimum Throttle Cutoff : simulink/Logic and Bit Operations/Compare To Constant  relop=>=  const=5  OutDataTypeStr=uint8
  Product : Product
  Product2 : Product  OutDataTypeStr=double
  Out5 : Outport
  wires:
  Minimum Throttle Cutoff/1 -> Product/2
  Product/1 -> Out5/1
  In5/1 -> Gain/1, Minimum Throttle Cutoff/1
  Gain/1 -> Product2/2
  Product2/1 -> Product/1
  Vs/1 -> Product2/1

== system phm_aug5_powertrain_r2018a/motorGroupTimMotors1/BLDC Motor4/throttle_fcn ==
  note: Output equals linearly scaled RPM
      | for given throttle input if throttle input >=Throttle Cuttoff (minThr)
      | else output is zero.
  In5 : Inport
  Vs : Inport  Port=2
  Gain : Gain  Gain=.01
  Minimum Throttle Cutoff : simulink/Logic and Bit Operations/Compare To Constant  relop=>=  const=5  OutDataTypeStr=uint8
  Product : Product
  Product2 : Product  OutDataTypeStr=double
  Out5 : Outport
  wires:
  Minimum Throttle Cutoff/1 -> Product/2
  Product/1 -> Out5/1
  In5/1 -> Gain/1, Minimum Throttle Cutoff/1
  Gain/1 -> Product2/2
  Product2/1 -> Product/1
  Vs/1 -> Product2/1

== system phm_aug5_powertrain_r2018a/motorGroupMarcosMotors1/motor1/motorRotor4/Electrical part ==
  Vin : Inport
  w angular speed : Inport  Port=2
  1/R : Gain  Gain=1/motorParams.Req
  Ke (Torque constant)1 : Gain  Gain=motorParams.Ke_eq
  Kt (Torque constant) Kt=Ke for an ideal square wave motor : Gain  Gain=motorParams.Ke_eq
  Sum : Sum  Inputs=|+-
  Electrical Torque : Outport
  current : Outport  Port=2
  wires:
  1/R/1 -> current/1, Kt (Torque constant) Kt=Ke for an ideal square wave motor/1  "current i"
  Sum/1 -> 1/R/1
  Kt (Torque constant) Kt=Ke for an ideal square wave motor/1 -> Electrical Torque/1
  Ke (Torque constant)1/1 -> Sum/2
  Vin/1 -> Sum/1
  w angular speed/1 -> Ke (Torque constant)1/1

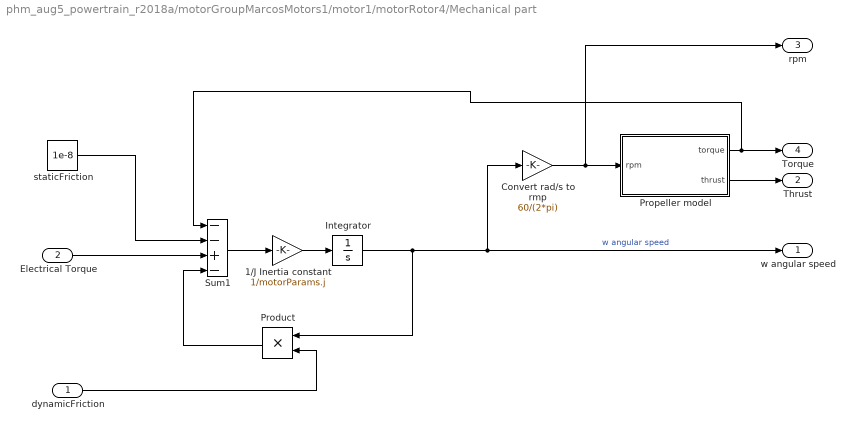
== system phm_aug5_powertrain_r2018a/motorGroupMarcosMotors1/motor1/motorRotor4/Mechanical part ==
  dynamicFriction : Inport
  Electrical Torque : Inport  Port=2
  1/J Inertia constant : Gain  Gain=1/motorParams.j
  Convert rad/s to rmp : Gain  Gain=60/(2*pi)
  Integrator : Integrator  InitialCondition=419
  Product : Product
  "Propeller model " : MATLAB Function  TreatAsAtomicUnit=on
  Sum1 : Sum  Inputs=--+-
  staticFriction : Constant  Value=1e-8
  w angular speed : Outport
  Thrust : Outport  Port=2
  rpm : Outport  Port=3
  Torque : Outport  Port=4
  wires:
  "Propeller model "/1(torque) -> Sum1/1, Torque/1
  1/J Inertia constant/1 -> Integrator/1
  dynamicFriction/1 -> Product/2
  Product/1 -> Sum1/4
  Integrator/1 -> Product/1, w angular speed/1, Convert rad/s to rmp/1  "w angular speed"
  Sum1/1 -> 1/J Inertia constant/1
  Electrical Torque/1 -> Sum1/3
  Convert rad/s to rmp/1 -> rpm/1, "Propeller model "/1(rpm)
  "Propeller model "/2(thrust) -> Thrust/1
  staticFriction/1 -> Sum1/2

== system phm_aug5_powertrain_r2018a/motorGroupMarcosMotors1/motor2/motorRotor4/Electrical part ==
  Vin : Inport
  w angular speed : Inport  Port=2
  1/R : Gain  Gain=1/motorParams.Req
  Ke (Torque constant)1 : Gain  Gain=motorParams.Ke_eq
  Kt (Torque constant) Kt=Ke for an ideal square wave motor : Gain  Gain=motorParams.Ke_eq
  Sum : Sum  Inputs=|+-
  Electrical Torque : Outport
  current : Outport  Port=2
  wires:
  1/R/1 -> current/1, Kt (Torque constant) Kt=Ke for an ideal square wave motor/1  "current i"
  Sum/1 -> 1/R/1
  Kt (Torque constant) Kt=Ke for an ideal square wave motor/1 -> Electrical Torque/1
  Ke (Torque constant)1/1 -> Sum/2
  Vin/1 -> Sum/1
  w angular speed/1 -> Ke (Torque constant)1/1

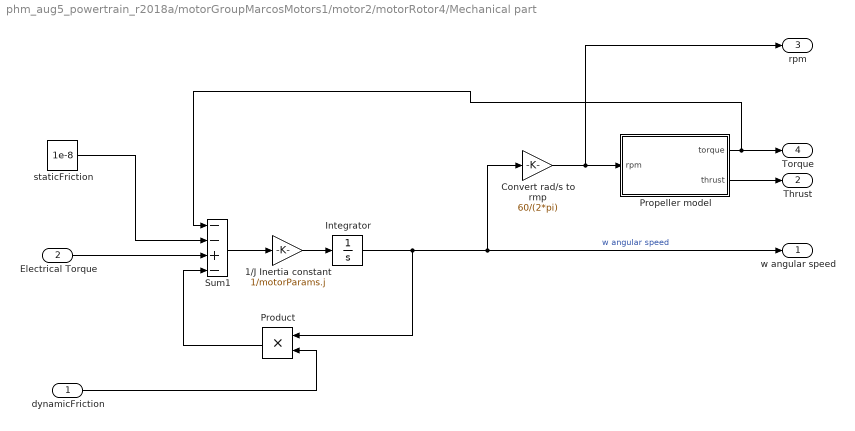
== system phm_aug5_powertrain_r2018a/motorGroupMarcosMotors1/motor2/motorRotor4/Mechanical part ==
  dynamicFriction : Inport
  Electrical Torque : Inport  Port=2
  1/J Inertia constant : Gain  Gain=1/motorParams.j
  Convert rad/s to rmp : Gain  Gain=60/(2*pi)
  Integrator : Integrator  InitialCondition=419
  Product : Product
  "Propeller model " : MATLAB Function  TreatAsAtomicUnit=on
  Sum1 : Sum  Inputs=--+-
  staticFriction : Constant  Value=1e-8
  w angular speed : Outport
  Thrust : Outport  Port=2
  rpm : Outport  Port=3
  Torque : Outport  Port=4
  wires:
  "Propeller model "/1(torque) -> Sum1/1, Torque/1
  1/J Inertia constant/1 -> Integrator/1
  dynamicFriction/1 -> Product/2
  Product/1 -> Sum1/4
  Integrator/1 -> Product/1, w angular speed/1, Convert rad/s to rmp/1  "w angular speed"
  Sum1/1 -> 1/J Inertia constant/1
  Electrical Torque/1 -> Sum1/3
  Convert rad/s to rmp/1 -> rpm/1, "Propeller model "/1(rpm)
  "Propeller model "/2(thrust) -> Thrust/1
  staticFriction/1 -> Sum1/2

== system phm_aug5_powertrain_r2018a/motorGroupMarcosMotors1/motor3/motorRotor4/Electrical part ==
  Vin : Inport
  w angular speed : Inport  Port=2
  1/R : Gain  Gain=1/motorParams.Req
  Ke (Torque constant)1 : Gain  Gain=motorParams.Ke_eq
  Kt (Torque constant) Kt=Ke for an ideal square wave motor : Gain  Gain=motorParams.Ke_eq
  Sum : Sum  Inputs=|+-
  Electrical Torque : Outport
  current : Outport  Port=2
  wires:
  1/R/1 -> current/1, Kt (Torque constant) Kt=Ke for an ideal square wave motor/1  "current i"
  Sum/1 -> 1/R/1
  Kt (Torque constant) Kt=Ke for an ideal square wave motor/1 -> Electrical Torque/1
  Ke (Torque constant)1/1 -> Sum/2
  Vin/1 -> Sum/1
  w angular speed/1 -> Ke (Torque constant)1/1

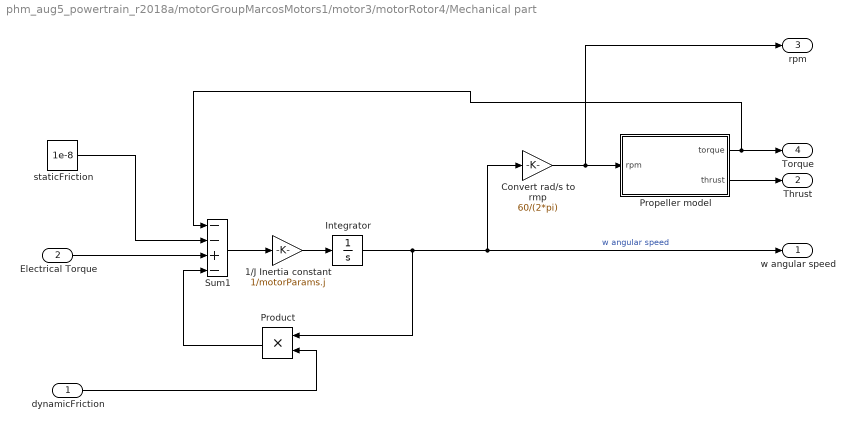
== system phm_aug5_powertrain_r2018a/motorGroupMarcosMotors1/motor3/motorRotor4/Mechanical part ==
  dynamicFriction : Inport
  Electrical Torque : Inport  Port=2
  1/J Inertia constant : Gain  Gain=1/motorParams.j
  Convert rad/s to rmp : Gain  Gain=60/(2*pi)
  Integrator : Integrator  InitialCondition=419
  Product : Product
  "Propeller model " : MATLAB Function  TreatAsAtomicUnit=on
  Sum1 : Sum  Inputs=--+-
  staticFriction : Constant  Value=1e-8
  w angular speed : Outport
  Thrust : Outport  Port=2
  rpm : Outport  Port=3
  Torque : Outport  Port=4
  wires:
  "Propeller model "/1(torque) -> Sum1/1, Torque/1
  1/J Inertia constant/1 -> Integrator/1
  dynamicFriction/1 -> Product/2
  Product/1 -> Sum1/4
  Integrator/1 -> Product/1, w angular speed/1, Convert rad/s to rmp/1  "w angular speed"
  Sum1/1 -> 1/J Inertia constant/1
  Electrical Torque/1 -> Sum1/3
  Convert rad/s to rmp/1 -> rpm/1, "Propeller model "/1(rpm)
  "Propeller model "/2(thrust) -> Thrust/1
  staticFriction/1 -> Sum1/2

== system phm_aug5_powertrain_r2018a/motorGroupMarcosMotors1/motor4/motorRotor4/Electrical part ==
  Vin : Inport
  w angular speed : Inport  Port=2
  1/R : Gain  Gain=1/motorParams.Req
  Ke (Torque constant)1 : Gain  Gain=motorParams.Ke_eq
  Kt (Torque constant) Kt=Ke for an ideal square wave motor : Gain  Gain=motorParams.Ke_eq
  Sum : Sum  Inputs=|+-
  Electrical Torque : Outport
  current : Outport  Port=2
  wires:
  1/R/1 -> current/1, Kt (Torque constant) Kt=Ke for an ideal square wave motor/1  "current i"
  Sum/1 -> 1/R/1
  Kt (Torque constant) Kt=Ke for an ideal square wave motor/1 -> Electrical Torque/1
  Ke (Torque constant)1/1 -> Sum/2
  Vin/1 -> Sum/1
  w angular speed/1 -> Ke (Torque constant)1/1

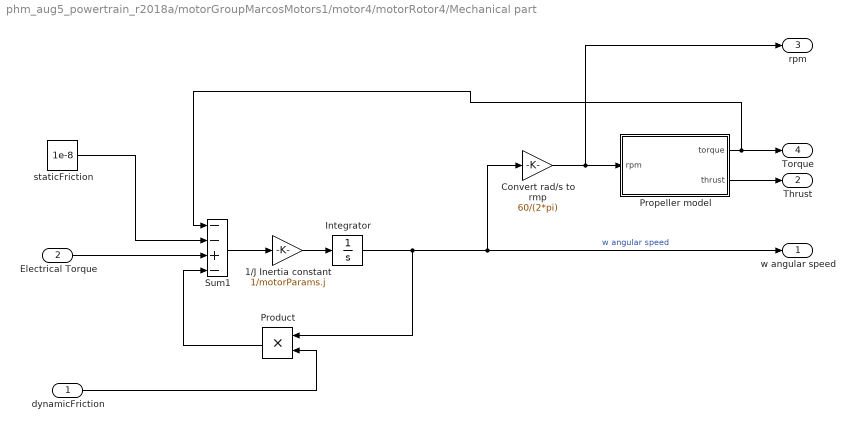
== system phm_aug5_powertrain_r2018a/motorGroupMarcosMotors1/motor4/motorRotor4/Mechanical part ==
  dynamicFriction : Inport
  Electrical Torque : Inport  Port=2
  1/J Inertia constant : Gain  Gain=1/motorParams.j
  Convert rad/s to rmp : Gain  Gain=60/(2*pi)
  Integrator : Integrator  InitialCondition=419
  Product : Product
  "Propeller model " : MATLAB Function  TreatAsAtomicUnit=on
  Sum1 : Sum  Inputs=--+-
  staticFriction : Constant  Value=1e-8
  w angular speed : Outport
  Thrust : Outport  Port=2
  rpm : Outport  Port=3
  Torque : Outport  Port=4
  wires:
  "Propeller model "/1(torque) -> Sum1/1, Torque/1
  1/J Inertia constant/1 -> Integrator/1
  dynamicFriction/1 -> Product/2
  Product/1 -> Sum1/4
  Integrator/1 -> Product/1, w angular speed/1, Convert rad/s to rmp/1  "w angular speed"
  Sum1/1 -> 1/J Inertia constant/1
  Electrical Torque/1 -> Sum1/3
  Convert rad/s to rmp/1 -> rpm/1, "Propeller model "/1(rpm)
  "Propeller model "/2(thrust) -> Thrust/1
  staticFriction/1 -> Sum1/2

== matlab function phm_aug5_powertrain_r2018a/Subsystem/MATLAB Function1 ==
  settings: updateMethod=DISCRETE  sampleTime=.2
  data: mu input; y output; sigma input
function y = addNoise(mu, sigma)

y = normrnd(mu, sigma);

== matlab function phm_aug5_powertrain_r2018a/Subsystem/MATLAB Function ==
  settings: updateMethod=DISCRETE  sampleTime=.2
  data: mu input; y output; sigma input
function y = addNoise(mu, sigma)

y = normrnd(mu, sigma);

== matlab function phm_aug5_powertrain_r2018a/motorGroupMarcosMotors1/motor1/motorRotor4/Mechanical part/Propeller model  ==
  data: torque output; rpm input; thrust output
function [torque,thrust] = fcn(rpm)
% angular_velocity in rpm

%coefficient of thrust, empirically derived
coef_t = 2*(10^-15)*rpm^3 - 4*(10^-11)*rpm^2 + 3*(10^-7)*rpm + .1013;
%thrust = coef_t * density of air * velocity^2 * propeller diameter (m) ^4
thrust = coef_t*1.225*(rpm/60)^2*.2^4;
% empirically derived
torque = 4*(10^-14)*rpm^3 +  8*(10^-12)*rpm^2 + 3*(10^-6)*rpm;
end

== matlab function phm_aug5_powertrain_r2018a/motorGroupMarcosMotors1/motor2/motorRotor4/Mechanical part/Propeller model  ==
  data: torque output; rpm input; thrust output
function [torque,thrust] = fcn(rpm)
% angular_velocity in rpm

%coefficient of thrust, empirically derived
coef_t = 2*(10^-15)*rpm^3 - 4*(10^-11)*rpm^2 + 3*(10^-7)*rpm + .1013;
%thrust = coef_t * density of air * velocity^2 * propeller diameter (m) ^4
thrust = coef_t*1.225*(rpm/60)^2*.2^4;
% empirically derived
torque = 4*(10^-14)*rpm^3 +  8*(10^-12)*rpm^2 + 3*(10^-6)*rpm;
end

== matlab function phm_aug5_powertrain_r2018a/motorGroupTimMotors1/BLDC Motor1/Propeller model  ==
  data: thrust output; torque output; rpm input
function [thrust,torque] = fcn(rpm)
% angular_velocity in rpm

%coefficient of thrust, empirically derived
coef_t = 2*(10^-15)*rpm^3 - 4*(10^-11)*rpm^2 + 3*(10^-7)*rpm + .1013;
%thrust = coef_t * density of air * velocity^2 * propeller diameter (m) ^4
thrust = coef_t*1.225*(rpm/60)^2*.2^4;
% empirically derived
torque = 4*(10^-14)*rpm^3 +  8*(10^-12)*rpm^2 + 3*(10^-6)*rpm;
end

== matlab function phm_aug5_powertrain_r2018a/motorGroupTimMotors1/BLDC Motor2/Propeller model  ==
  data: thrust output; torque output; rpm input
function [thrust,torque] = fcn(rpm)
% angular_velocity in rpm

%coefficient of thrust, empirically derived
coef_t = 2*(10^-15)*rpm^3 - 4*(10^-11)*rpm^2 + 3*(10^-7)*rpm + .1013;
%thrust = coef_t * density of air * velocity^2 * propeller diameter (m) ^4
thrust = coef_t*1.225*(rpm/60)^2*.2^4;
% empirically derived
torque = 4*(10^-14)*rpm^3 +  8*(10^-12)*rpm^2 + 3*(10^-6)*rpm;
end

== matlab function phm_aug5_powertrain_r2018a/motorGroupTimMotors1/BLDC Motor3/Propeller model  ==
  data: thrust output; torque output; rpm input
function [thrust,torque] = fcn(rpm)
% angular_velocity in rpm

%coefficient of thrust, empirically derived
coef_t = 2*(10^-15)*rpm^3 - 4*(10^-11)*rpm^2 + 3*(10^-7)*rpm + .1013;
%thrust = coef_t * density of air * velocity^2 * propeller diameter (m) ^4
thrust = coef_t*1.225*(rpm/60)^2*.2^4;
% empirically derived
torque = 4*(10^-14)*rpm^3 +  8*(10^-12)*rpm^2 + 3*(10^-6)*rpm;
end

== matlab function phm_aug5_powertrain_r2018a/motorGroupTimMotors1/BLDC Motor4/Propeller model  ==
  data: thrust output; torque output; rpm input
function [thrust,torque] = fcn(rpm)
% angular_velocity in rpm

%coefficient of thrust, empirically derived
coef_t = 2*(10^-15)*rpm^3 - 4*(10^-11)*rpm^2 + 3*(10^-7)*rpm + .1013;
%thrust = coef_t * density of air * velocity^2 * propeller diameter (m) ^4
thrust = coef_t*1.225*(rpm/60)^2*.2^4;
% empirically derived
torque = 4*(10^-14)*rpm^3 +  8*(10^-12)*rpm^2 + 3*(10^-6)*rpm;
end

== matlab function phm_aug5_powertrain_r2018a/motorGroupMarcosMotors1/motor3/motorRotor4/Mechanical part/Propeller model  ==
  data: torque output; rpm input; thrust output
function [torque,thrust] = fcn(rpm)
% angular_velocity in rpm

%coefficient of thrust, empirically derived
coef_t = 2*(10^-15)*rpm^3 - 4*(10^-11)*rpm^2 + 3*(10^-7)*rpm + .1013;
%thrust = coef_t * density of air * velocity^2 * propeller diameter (m) ^4
thrust = coef_t*1.225*(rpm/60)^2*.2^4;
% empirically derived
torque = 4*(10^-14)*rpm^3 +  8*(10^-12)*rpm^2 + 3*(10^-6)*rpm;
end

== matlab function phm_aug5_powertrain_r2018a/motorGroupMarcosMotors1/motor4/motorRotor4/Mechanical part/Propeller model  ==
  data: torque output; rpm input; thrust output
function [torque,thrust] = fcn(rpm)
% angular_velocity in rpm

%coefficient of thrust, empirically derived
coef_t = 2*(10^-15)*rpm^3 - 4*(10^-11)*rpm^2 + 3*(10^-7)*rpm + .1013;
%thrust = coef_t * density of air * velocity^2 * propeller diameter (m) ^4
thrust = coef_t*1.225*(rpm/60)^2*.2^4;
% empirically derived
torque = 4*(10^-14)*rpm^3 +  8*(10^-12)*rpm^2 + 3*(10^-6)*rpm;
end
